simulink model "ACC_RRScen_RTMaps_CoSim"  (R2024a)
settings: Solver=FixedStepAuto  StartTime=0  StopTime=100  FixedStep=0.05  RelTol=1e-3
undefined symbols (not defined in the file): Defined, driverSetSpeed, Ego, Lane, m, matlabshared, simStepSize, User
libraries: roadrunnerscenario x4, hostiolib x2, drivingscenarioandsensors x1, autolibshared x1
settings Model: Creator=darkh  LastModifiedBy=darkh

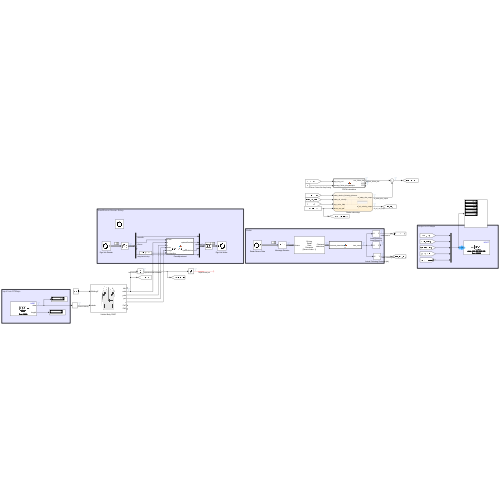
[thumbnail: Simulink's stored preview of the top-level diagram]
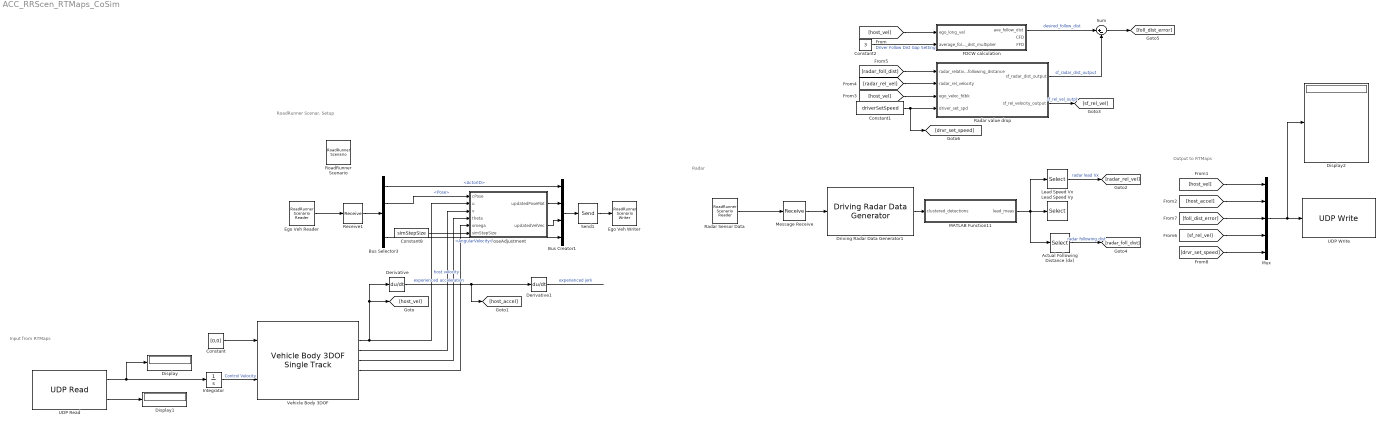
== system ACC_RRScen_RTMaps_CoSim ==
  note: Input from RTMaps
  note: Output to RTMaps
  note: RoadRunner Scenar. Setup
  note: Radar
  Actual Following Distance (dx) : Selector  InputPortWidth=6  IndexOptions=Index vector (dialog)  Indices=[1]  OutputSizes=1
  Bus Creator1 : BusCreator  Inputs=4  OutDataTypeStr=Bus: BusActorRuntime  NonVirtualBus=on
      settings: InheritFromInputs=off
  Bus Selector3 : BusSelector  OutputSignals=ActorID,Pose,Velocity,AngularVelocity
  Constant : Constant  Value=[0,0]
  Constant1 : Constant  Value=driverSetSpeed
  Constant2 : Constant  Value=3
  Constant8 : Constant  Value=simStepSize
  Derivative : Derivative
  Derivative1 : Derivative
  Display : Display
  Display1 : Display
  Display2 : Display
  Driving Radar Data Generator1 : drivingscenarioandsensors/Driving Radar Data Generator  SensorIndex=1  UpdateRate=20  MountingLocation=[ 3.4, 0, 0.2 ]  MountingAngles=[0 0 0]  HasElevation=off  HasRangeRate=on  HasNoise=off  HasFalseAlarms=off  HasOcclusion=on  MaxNumReportsSource=Property  MaxNumReports=50  TargetReportFormat=Clustered detections  DetectionCoordinates=Body  TrackCoordinates=Body  BusNameSource=Auto  BusName=BusDrivingRadarDataGenerator  AzimuthResolution=4  ElevationResolution=5  RangeResolution=2.5  RangeRateResolution=0.5  AzimuthBiasFraction=0.1  ElevationBiasFraction=0.1  RangeBiasFraction=0.05  RangeRateBiasFraction=0.05  FieldOfView=[ 20, 5 ]  RangeLimits=[ 0, 150 ]  RangeRateLimits=[ -100, 100 ]  DetectionProbability=0.9  FalseAlarmRate=1e-06  ReferenceRange=100  ReferenceRCS=0  CenterFrequency=77e9  FilterInitializationFcn=initcvekf  ConfirmationThreshold=[2 3]  DeletionThreshold=[5 5]  InitialSeedSource=Repeatable  InitialSeed=0  UsedSeed=matlabshared.tracking.internal.SimulinkUtilities.seedManager(gcb)  ProfilesSource=From Scenario Reader block  ProfilesParameters=driving.internal.ActorProfilesRadarParameters  ProfilesExpression=struct('ClassID',0,'Length',4.7,'Width',1.8,'Height',1.4,'OriginOffset',[-1.35 0 0],'RCSPattern',[10 10;10 10],'RCSAzimuthAngles',[-180 180],'RCSElevationAngles',[-90 90])
  Ego Veh Reader : roadrunnerscenario/RoadRunner Scenario Reader  TopicCategory=Actor  ActorCategory=All Types  ActionType=Path Following  EventType=User-Defined  TopicType=Actor Pose  VehicleType=Vehicle Specifications  UserDefinedAction=Action1  UserDefinedEvent=Event1  Filter=Self  SensorTopic=Target Poses  LaneBoundaryOutputTopic=Ego-Lane  SensorID=1  SampleTime=simStepSize
  Ego Veh Writer : roadrunnerscenario/RoadRunner Scenario Writer  TopicCategory=Actor  ActorCategory=All Types  EventType=Action Complete  UserDefinedEvent=Event1  VehicleType=Vehicle Pose  TopicType=Actor Pose
  FDCW calculation : MATLAB Function  TreatAsAtomicUnit=on
  Integrator : Integrator
  Lead Speed Vx : Selector  InputPortWidth=6  IndexOptions=Index vector (dialog)  Indices=4  OutputSizes=1
  Lead Speed Vy : Selector  InputPortWidth=6  IndexOptions=Index vector (dialog)  Indices=5  OutputSizes=1
  MATLAB Function11 : MATLAB Function  TreatAsAtomicUnit=on
  Message Receive : Receive  InputPortMessageModes=m  UseInternalQueue=off
  Mux : Mux  Inputs=5
  PoseAdjustment : MATLAB Function  TreatAsAtomicUnit=on
  Radar Sensor Data : roadrunnerscenario/RoadRunner Scenario Reader  TopicCategory=Sensor  ActorCategory=All Types  ActionType=Path Following  EventType=User-Defined  TopicType=Actor Specifications  VehicleType=Vehicle Specifications  UserDefinedAction=Action1  UserDefinedEvent=Event1  Filter=Self  SensorTopic=Target Poses  LaneBoundaryOutputTopic=Ego-Lane  SensorID=1  SampleTime=simStepSize
  Radar value drop : Stateflow chart  TreatAsAtomicUnit=on
  Receive1 : Receive  InputPortMessageModes=m  UseInternalQueue=off  QueueOverwriting=on  QueueLength=1  QueueType=LIFO
  RoadRunner Scenario : roadrunnerscenario/RoadRunner Scenario  UserDefinedActions={}  UserDefinedEvents={}
  Send1 : Send  OutputPortMessageModes=m
  Sum : Sum  Inputs=|+-
  UDP Read : hostiolib/UDP Read  localURL='0.0.0.0'  localPort=9999  remoteURL='0.0.0.0'  remotePort=-1  recvBufferSize=8192  dims=1  signalDatatype=double  isVarSize=off  showBlockingTime=on  blockingTime=0  sampletime=simStepSize  blockPlatform=HOST  hoistedMaskSrc=UDP Read/UDP Read Sim/UDP Read
  UDP Write : hostiolib/UDP Write  remoteURL='255.255.255.255'  remotePort=25000  localURL='255.255.255.255'  localPortSource=Automatically determine  localPort=-1  sampletime=-1  separateLengthPort=0  blockPlatform=HOST  hoistedMaskSrc=UDP Write/UDP Write Sim/UDP Write
  "Vehicle Body 3DOF " : autolibshared/Vehicle Body 3DOF Single Track  trackMode=Dual  inputMode=External longitudinal velocity  frontSteerMode=on  rearSteerMode=off  windMode=off  muMode=off  extFMode=off  extMMode=off  htchFMode=off  htchMMode=off  extXo=off  extpsio=off  extxdoto=off  extro=off  extYo=off  extTamb=off  extydoto=off  aMode=2  NF=2  NR=2  m=m  a=1.5569  b=1.5371  h=0.18903  dh=1  hh=0.2  X_o=0  xdot_o=0  CalphaMode=off  sigmaMode=on  d=0  hl=0  w=[1.4,1.4]  Cy_f=40000  Cy_r=40000  sigma_f=.1  sigma_r=.1  alpha_f_brk=[-.1 .1]  Cy_f_data=[-9e3 9e3]  alpha_r_brk=[-.1 .1]  Cy_r_data=[-9e3 9e3]  Y_o=0  ydot_o=0  Izz=2066  psi_o=0  r_o=0  Af=2.73  Cd=.30356  Cl=.1  Cpm=.1  beta_w=[0 0.01:0.01:0.3]  Cs=[0 0.01:0.01:0.3]  Cym=[0 1e-6:0.01:0.3]  Pabs=101325  Tair=273  g=9.81  mu=1  xdot_tol=.01  Fznom=5000  Fxtire_sat=7e4  Fytire_sat=7e4  longOff=0  latOff=0  vertOff=0  wrapAng=off
  wires:
  Constant8/1 -> PoseAdjustment/6(simStepSize)
  Send1/1 -> Ego Veh Writer/1
  "Vehicle Body 3DOF "/2 -> PoseAdjustment/2(u), [host_vel], Derivative/1  "host velocity"
  Ego Veh Reader/1 -> Receive1/1
  Bus Creator1/1 -> Send1/1
  Radar Sensor Data/1 -> Message Receive/1
  PoseAdjustment/2(updatedVelVec) -> Bus Creator1/3
  Bus Selector3/1 -> Bus Creator1/1  "<ActorID>"
  Bus Selector3/4 -> Bus Creator1/4  "<AngularVelocity>"
  PoseAdjustment/1(updatedPoseMat) -> Bus Creator1/2
  Integrator/1 -> "Vehicle Body 3DOF "/2  "Control Velocity"
  Bus Selector3/2 -> PoseAdjustment/1(cPose)  "<Pose>"
  Receive1/1 -> Bus Selector3/1
  Driving Radar Data Generator1/1 -> MATLAB Function11/1(clustered_detections)
  Constant/1 -> "Vehicle Body 3DOF "/1
  Derivative1/1 -> ?  "experienced jerk"
  Message Receive/1 -> Driving Radar Data Generator1/1
  MATLAB Function11/1(lead_meas) -> Actual Following Distance (dx)/1, Lead Speed Vy/1, Lead Speed Vx/1
  Derivative/1 -> [host_accel], Derivative1/1  "experienced acceleration"
  "Vehicle Body 3DOF "/5 -> PoseAdjustment/5(omega)
  "Vehicle Body 3DOF "/3 -> PoseAdjustment/3(v)
  "Vehicle Body 3DOF "/4 -> PoseAdjustment/4(theta)
  UDP Read/1 -> Display/1, Integrator/1
  UDP Read/2 -> Display1/1
  [host_vel] -> FDCW calculation/1(ego_long_vel)
  Mux/1 -> Display2/1, UDP Write/1
  [host_vel] -> Radar value drop/3(ego_veloc_fdbk)
  Lead Speed Vx/1 -> [radar_rel_vel]  "radar lead Vx"
  [radar_rel_vel] -> Radar value drop/2(radar_rel_velocity)
  Radar value drop/2(sf_rel_velocity_output) -> [sf_rel_vel]  "sf_rel_vel_outpt"
  FDCW calculation/1(ave_follow_dist) -> Sum/1  "desired_follow_dist"
  Actual Following Distance (dx)/1 -> [radar_foll_dist]  "radar following dist"
  [radar_foll_dist] -> Radar value drop/1(radar_relative_following_distance)
  Radar value drop/1(sf_radar_dist_output) -> Sum/2  "sf_radar_dist_output"
  Sum/1 -> [foll_dist_error]
  Constant1/1 -> [drvr_set_speed], Radar value drop/4(driver_set_spd)
  [host_vel] -> Mux/1
  [foll_dist_error] -> Mux/3
  [host_accel] -> Mux/2
  [sf_rel_vel] -> Mux/4
  [drvr_set_speed] -> Mux/5
  Constant2/1 -> FDCW calculation/2(average_follow_dist_multiplier)  "Driver Follow Dist Gap Setting"

== stateflow chart ACC_RRScen_RTMaps_CoSim/Radar value drop ==
  state Radar_State_Lead_Veh_Present_and_Detected
    sf_radar_dist_output = radar_relative_following_distance;
    % sf_radar_dist_output = smooth_switch(sf_radar_dist_output, radar_relative_following_distance, 0.05, 2);
    sf_rel_velocity_output = radar_rel_velocity;
    %sf_rel_velocity_output = smooth_switch(sf_rel_velocity_output, radar_rel_velocity, 0.05, 1);
  state Output_Spoof_To_Keep_Moving
    % sf_radar_dist_output = 150;
    sf_radar_dist_output = smooth_switch(sf_radar_dist_output, 150, 0.05, 2);
    set_spd_err = driver_set_spd - ego_veloc_fdbk;
    % sf_rel_velocity_output = set_spd_err;
    sf_rel_velocity_output = smooth_switch(sf_rel_velocity_output, set_spd_err, 0.05, 5);
  (default) -> Radar_State_Lead_Veh_Present_and_Detected : {sf_radar_dist_output = radar_relative_following_distance;
      | sf_rel_velocity_output = radar_rel_velocity;}
  Radar_State_Lead_Veh_Present_and_Detected -> Output_Spoof_To_Keep_Moving : [radar_relative_following_distance == 0 && radar_rel_velocity < 0.9]
  Output_Spoof_To_Keep_Moving -> Radar_State_Lead_Veh_Present_and_Detected : [radar_relative_following_distance > 0]
  data: prev_val function_input; curr_val function_input; dt function_input; tau function_input; filtered_val function_output; radar_relative_following_distance input; sf_radar_dist_output output; radar_rel_velocity input; ego_veloc_fdbk input; sf_rel_velocity_output output; driver_set_spd input; set_spd_err local
  function filtered_val = smooth_switch(prev_val, curr_val, dt, tau):
    | function filtered_val = smooth_switch(prev_val, curr_val, dt, tau)
    | % Smooth transition from prev_val toward curr_val
    | % dt  = sample time [s]; equal to system sample time of 0.05s currently
    | % tau = time constant [s] (0.3–1.0 typical)
    | 
    | if isempty(prev_val)
    |     prev_val = 0;
    | end
    | 
    | alpha = exp(-dt/tau);
    | filtered_val = alpha*prev_val + (1-alpha)*curr_val;
    | end

== matlab function ACC_RRScen_RTMaps_CoSim/PoseAdjustment ==
  data: cPose input; u input; updatedPoseMat output; v input; theta input; omega input; updatedVelVec output; simStepSize input
function [updatedPoseMat, updatedVelVec] = RRPoseAdjustment(cPose, u, v, theta, omega, simStepSize)
    thetad = theta + omega*simStepSize;
    xd = (u*cos(theta) - v*sin(theta))*simStepSize;
    yd = (u*sin(theta) + v*cos(theta))*simStepSize;
    pose_mat = [cos(-thetad) -sin(-thetad) 0 (yd+cPose(1,4)); sin(-thetad) cos(-thetad) 0 (xd+cPose(2,4)); 0 0 1 0; 0 0 0 1];
    updatedPoseMat = pose_mat;
    updatedVelVec = [u*sin(theta) + v*cos(theta), u*cos(theta) - v*sin(theta), 0];
    return;
end

== matlab function ACC_RRScen_RTMaps_CoSim/MATLAB Function11 ==
  data: clustered_detections input Bus: BusRadar; lead_meas output double
function lead_meas = fcn(clustered_detections)

lead_det = clustered_detections.Detections(1);
lead_meas = lead_det.Measurement;

% relative_dist = sqrt(lead_det.Measurement(1)^2 + lead_det.Measurement(2)^2); % rel_dist = sqrt(x^2+y^2)
% relative_speed = sqrt(lead_det.Measurement(4)^2 + lead_det.Measurement(5)^2);
end

== matlab function ACC_RRScen_RTMaps_CoSim/FDCW calculation ==
  settings: updateMethod=DISCRETE
  data: ego_long_vel input; ave_follow_dist output; CFD output; FFD output; average_follow_dist_multiplier input
% Function to determine the closest (CFD) and furthest follow distance (FFD) for the
% ego vehicle relative to the lead vehicle given the ego vehicle's current
% velocity

% This function outputs the middle distance value between the CFD and FFD
% and those values respectively as well

function [ave_follow_dist, CFD, FFD] = fcn(ego_long_vel, average_follow_dist_multiplier)
    persistent dist_history window_size smoothing_weights
    
    % Initialize (first call only)
    if isempty(dist_history)
        window_size = 5;  % Number of past samples
        dist_history = zeros(1, window_size);
        
        % Define and normalize weights (e.g., linear decay)
        smoothing_weights = linspace(1, 0.5, window_size);  % Weights from 1.0 to 0.5
        smoothing_weights = smoothing_weights / sum(smoothing_weights);  % Normalize
    end
    ego_long_vel_mph = ego_long_vel*2.23694;
    
    if ego_long_vel_mph > 0 && ego_long_vel_mph < 20
        CFD = 2.8*ego_long_vel_mph^0.45+8;
        FFD = 100-0.2*(20-ego_long_vel_mph)^2;
    elseif ego_long_vel_mph <= 0
        CFD = 8;
        FFD = 100-0.2*(20)^2;
    else
        CFD = 2.8*ego_long_vel_mph^0.45+8;
        FFD = 100;
    end
    % AveFollowDist_Gain = 3;
    AveFollowDist_Gain = average_follow_dist_multiplier;

    % --- Update history buffer ---
    dist_history = [ ((AveFollowDist_Gain-1)*CFD + FFD)/AveFollowDist_Gain , dist_history(1:end-1)];  % FIFO

    % --- Smoothed average (weighted, normalized) ---
    smoothed_ave_dist = sum(dist_history .* smoothing_weights);
    
    % --- Clamp to CFD/FFD bounds ---
    ave_follow_dist = min(max(smoothed_ave_dist, CFD), FFD);
end
